simulink model "linear_without_RW"  (R2024b)
settings: Solver=VariableStepAuto  StartTime=0.0  StopTime=10.0  RelTol=1e-3
settings Model: Creator=bedag  LastModifiedBy=bedag

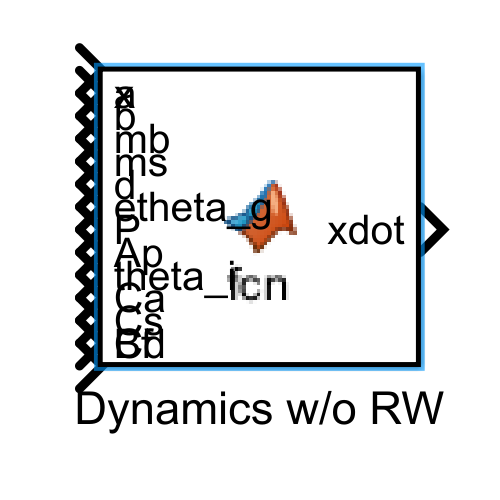
[thumbnail: Simulink's stored preview of the top-level diagram]
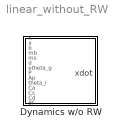
== system linear_without_RW ==
  Dynamics w/o RW : MATLAB Function  TreatAsAtomicUnit=on

== matlab function linear_without_RW/Dynamics w//o RW ==
  data: x input; a input; b input; mb input; ms input; d input; etheta_g input; xdot output; P input; Ap input; theta_i input; Ca input; Cs input; Cd input; Bf input
function xdot = fcn(x, a, b, mb, ms, d, etheta_g, P, Ap, theta_i, Ca, Cs, Cd, Bf)

xt = b*mb*sin(theta_g)/(mb+ms);
zt = (b*mb*cos(theta_g) + d*mb + (d-e)*ms)/(mb+ms);
l = a/(3*cos(theta_i)); 

alpha = x(1);
beta = x(2);
gamma = x(3);

dtxdg = 2*P*Ap*zt*cos(theta_i)*sin(beta)*cos(gamma)...
        * (2*(Ca+2*Cs*sin(theta_i)^2+Cd)*cos(beta)...
        + Bf*Cd*sin(theta_i)*tan(theta_i))...
        - 2*P*Ap*l*sin(theta_i)*sin(beta)*cos(gamma)...
        * ((3*Ca+4*Cs+3*Cd)*cos(theta_i)*cos(beta)+Bf*Cd);

dtydb = 4*P*Ap*xt*cos(theta_i)...
        * (-2*cos(beta)*sin(beta)*(Ca+Cs*(-3*sin(theta_i)^2+2)+Cd)...
        - Bf*Cd*cos(theta_i)*sin(beta)+Cs*sin(theta_i)^2)...
        + 2*P*Ap*zt*cos(theta_i)*cos(beta)*cos(gamma)*Bf*Cd*sin(theta_i)*tan(theta_i)...
        + 2*P*Ap*zt*cos(theta_i)*cos(beta)*cos(gamma)*(2*(Ca+2*Cs*sin(theta_i)^2+Cd)*cos(beta))...
        - 2*P*Ap*zt*cos(theta_i)*sin(beta)*cos(gamma)*(2*(Ca+2*Cs*sin(theta_i)^2+Cd)*sin(beta))...
        - 2*P*Ap*l*sin(theta_i)*cos(beta)*cos(gamma)*((3*Ca+4*Cs+3*Cd)*cos(theta_i)*cos(beta))...
        + 2*P*Ap*l*sin(theta_i)*sin(beta)*cos(gamma)*((3*Ca+4*Cs+3*Cd)*cos(theta_i)*sin(beta))...
        - 2*P*Ap*l*sin(theta_i)*sin(beta)*cos(gamma)*Bf*Cd;

dtzdg = 2*P*Ap*xt*sin(beta)*cos(gamma)*(-2*(Ca+2*Cs*sin(theta_i)^2+Cd)*cos(theta_i)*cos(beta)-Bf*Cd*sin(theta_i)^2);

A11 = zeros(3,3);
A12 = eye(3);
A21 = [-1/sin(beta) 0 0; 
       0 1 0;
       1/tan(beta) 0 1]/I*[0 0 dtxdg; 0 dtydb 0; 0 0 dtzdg];
A22 = zeros(3,3);

A = [A11 A12; A21 A22];

xdot = A*x;
